simulink model "vikramsolarboost"  (R2017a)
settings: Solver=VariableStepAuto  StartTime=0.0  StopTime=1  MaxStep=1e-4  RelTol=1e-3
libraries: powerlib x11, powerlib_extras x2, simulink x2, powerlib_meascontrol x1
settings Model: Creator=Ankita Arora  LastModifiedBy=2
settings SolverCC: ZeroCrossAlgorithm=Adaptive
settings OptimizationCC: LifeSpan=inf
settings DebuggingCC: SFExecutionAtInitializationDiag=none

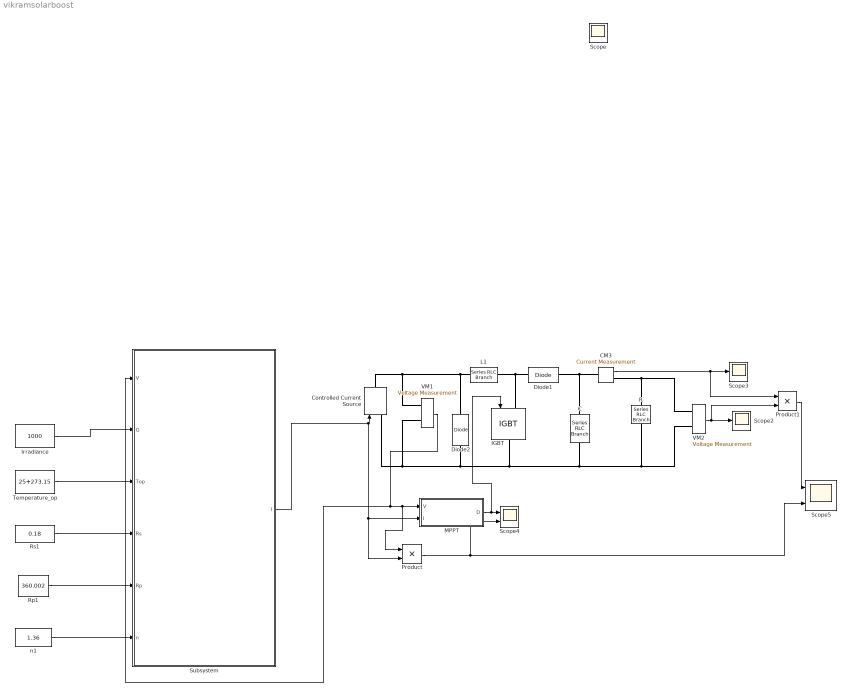
== system vikramsolarboost ==
  C : powerlib/Elements/Series RLC Branch  LConnTagsString=__new0  RConnTagsString=__new0  BranchType=C  Resistance=0.01  Inductance=1.0  SetiL0=off  InitialCurrent=0  Capacitance=3e-03  Setx0=off  InitialVoltage=200  Measurements=None
  CM3 : powerlib/Measurements/Current Measurement  Tag=PoWeRsYsTeMmEaSuReMeNt  PhasorSimulation=off  OutputType=Magnitude  PSBequivalent=0
  Controlled Current Source : powerlib/Electrical Sources/Controlled Current Source  Initialize=on  Source_Type=AC  Amplitude=0  Phase=0  Frequency=0  Measurements=None
  Diode1 : powerlib/Power Electronics/Diode  Ron=0.001  Lon=0  Vf=0.8  IC=0  UseSnubber=off  Rs=500  Cs=250e-9  Measurements=off
  Diode2 : powerlib/Power Electronics/Diode  Ron=0.001  Lon=0  Vf=0.8  IC=0  UseSnubber=off  Rs=500  Cs=250e-9  Measurements=off
  IGBT : powerlib/Power Electronics/IGBT  Ron=0.001  Lon=0  Vf=1  Tf=1e-6  Tt=2e-6  IC=0  Rs=1e5  Cs=inf  Measurements=off
  Irradiance : Constant  Value=1000
  L1 : powerlib/Elements/Series RLC Branch  LConnTagsString=__new0  RConnTagsString=__new0  BranchType=L  Resistance=1.0  Inductance=8.5e-03  SetiL0=off  InitialCurrent=0  Capacitance=1.0  Setx0=off  InitialVoltage=0  Measurements=None
  MPPT : Subsystem
  Product : Product  RndMeth=Zero
  Product1 : Product  RndMeth=Zero
  R : powerlib/Elements/Series RLC Branch  LConnTagsString=__new0  RConnTagsString=__new0  BranchType=R  Resistance=40  Inductance=1.0  SetiL0=off  InitialCurrent=0  Capacitance=1.0  Setx0=off  InitialVoltage=0  Measurements=None
  Rp1 : Constant  Value=360.002
  Rs1 : Constant  Value=0.18
  Scope : Scope
  Scope2 : Scope
  Scope3 : Scope
  Scope4 : Scope  NumInputPorts=2
  Scope5 : Scope  NumInputPorts=2
  Subsystem : Subsystem
  Temperature_op : Constant  Value=25+273.15
  VM1 : powerlib/Measurements/Voltage Measurement  Tag=PoWeRsYsTeMmEaSuReMeNt  PhasorSimulation=off  OutputType=Magnitude  PSBequivalent=0
  VM2 : powerlib/Measurements/Voltage Measurement  Tag=PoWeRsYsTeMmEaSuReMeNt  PhasorSimulation=off  OutputType=Magnitude  PSBequivalent=0
  n1 : Constant  Value=1.36
  wires:
  Temperature_op/1 -> Subsystem/3(Top)
  Rs1/1 -> Subsystem/4(Rs)
  Rp1/1 -> Subsystem/5(Rp)
  n1/1 -> Subsystem/6(n)
  CM3/1 -> Product1/1, Scope3/1
  VM2/1 -> Product1/2, Scope2/1
  Product/1 -> Scope5/2, Scope4/2
  MPPT/1(D) -> IGBT/1, Scope4/1
  Subsystem/1(I) -> MPPT/2(I), Product/2, Controlled Current Source/1
  Product1/1 -> Scope5/1
  VM1/1 -> Product/1, MPPT/1(V), Subsystem/1(V)
  Irradiance/1 -> Subsystem/2(G)
  connections:
  C/RConn1 -- VM2/LConn2 -- R/RConn1 -- IGBT/RConn1 -- Diode2/LConn1 -- Controlled Current Source/LConn1 -- VM1/LConn2
  Diode1/RConn1 -- CM3/LConn1 -- C/LConn1
  IGBT/LConn1 -- L1/RConn1 -- Diode1/LConn1
  VM2/LConn1 -- R/LConn1 -- CM3/RConn1
  VM1/LConn1 -- Diode2/RConn1 -- L1/LConn1 -- Controlled Current Source/RConn1

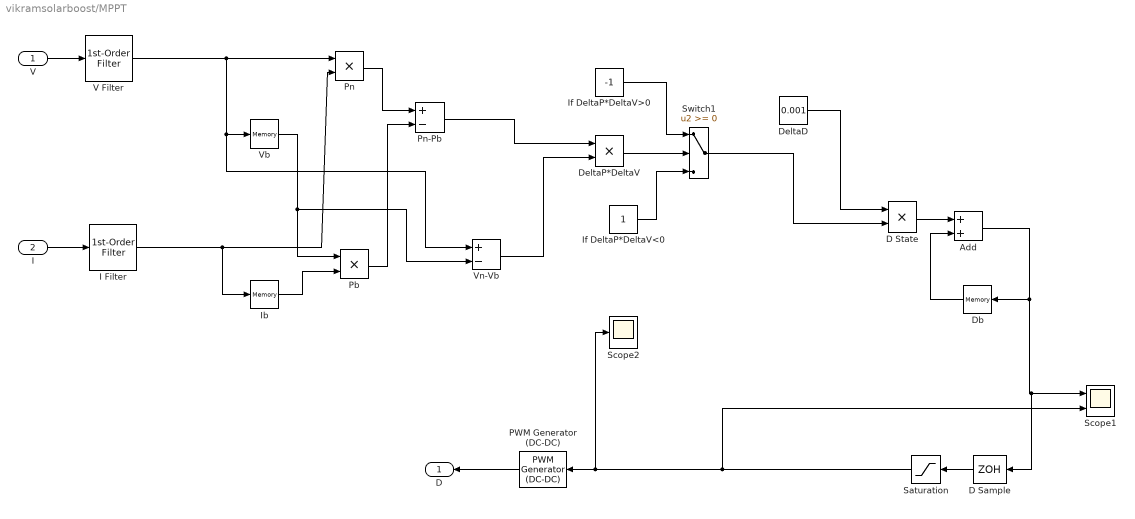
== system vikramsolarboost/MPPT ==
  V : Inport
  I : Inport  Port=2
  Add : Sum
  D Sample : ZeroOrderHold  SampleTime=1e-4
  D State : Product  RndMeth=Zero
  Db : Memory  InheritSampleTime=on  LinearizeAsDelay=on
  DeltaD : Constant  Value=0.001
  DeltaP*DeltaV : Product  RndMeth=Zero
  I Filter : powerlib_extras/Control  Blocks/1st-Order  Filter  FilterType=Lowpass  Tc=1e-3  Initialize=off  Vac_Init=[0.8 -25 60]  Vdc_Init=-0.4  PlotResponse=off  param1=[1 500 1]
  Ib : Memory  InheritSampleTime=on  LinearizeAsDelay=on
  If DeltaP*DeltaV<0 : Constant
  If DeltaP*DeltaV>0 : Constant  Value=-1
  PWM Generator (DC-DC) : powerlib_meascontrol/Pulse & Signal Generators/PWM Generator (DC-DC)  Fsw=5000  Ts=0
  Pb : Product  RndMeth=Zero
  Pn : Product  RndMeth=Zero
  Pn-Pb : Sum  Inputs=+-
  Saturation : Saturate  UpperLimit=0.8  LowerLimit=0
  Scope1 : Scope  NumInputPorts=2
  Scope2 : Scope
  Switch1 : Switch
  V Filter : powerlib_extras/Control  Blocks/1st-Order  Filter  FilterType=Lowpass  Tc=1e-3  Initialize=off  Vac_Init=[0.8 -25 60]  Vdc_Init=-0.4  PlotResponse=off  param1=[1 500 1]
  Vb : Memory  InheritSampleTime=on  LinearizeAsDelay=on
  Vn-Vb : Sum  Inputs=+-
  D : Outport
  wires:
  V/1 -> V Filter/1
  I/1 -> I Filter/1
  I Filter/1 -> Ib/1, Pn/2
  V Filter/1 -> Pn/1, Vb/1, Vn-Vb/1
  Ib/1 -> Pb/2
  Vb/1 -> Pb/1, Vn-Vb/2
  Pn/1 -> Pn-Pb/1
  Pb/1 -> Pn-Pb/2
  D State/1 -> Add/1
  Db/1 -> Add/2
  Pn-Pb/1 -> DeltaP*DeltaV/1
  Vn-Vb/1 -> DeltaP*DeltaV/2
  DeltaP*DeltaV/1 -> Switch1/2
  If DeltaP*DeltaV>0/1 -> Switch1/1
  If DeltaP*DeltaV<0/1 -> Switch1/3
  Switch1/1 -> D State/2
  DeltaD/1 -> D State/1
  Add/1 -> Db/1, D Sample/1, Scope1/1
  PWM Generator (DC-DC)/1 -> D/1
  Saturation/1 -> Scope1/2, PWM Generator (DC-DC)/1, Scope2/1
  D Sample/1 -> Saturation/1

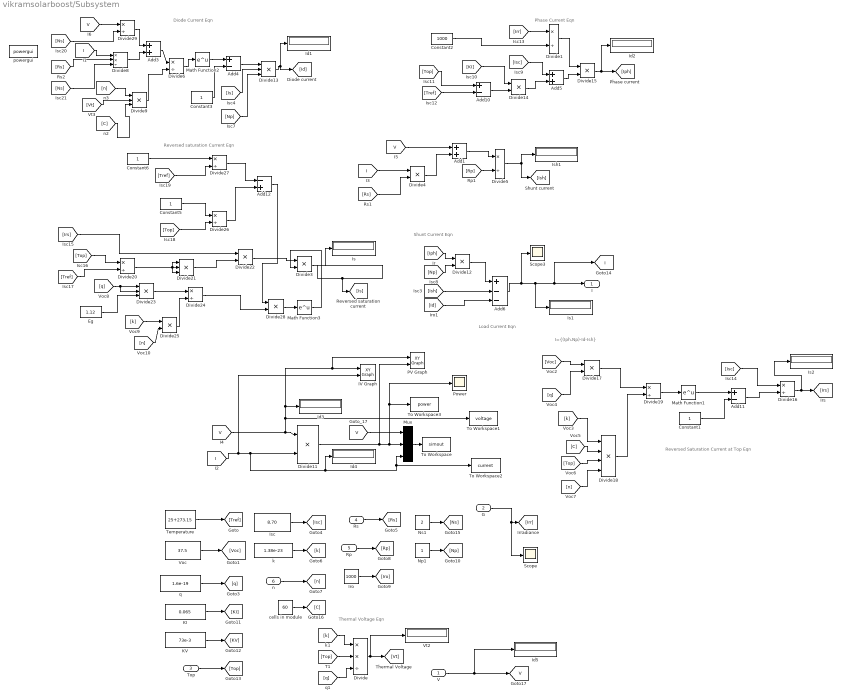
== system vikramsolarboost/Subsystem ==
  note: Diode Current Eqn
  note: Shunt Current Eqn
  note: Phase Current Eqn
  note: Reversed saturation Current Eqn
  note: Load Current Eqn
  note: I={(Iph.Np)-Id-Ish}
  note: Reversed Saturation Current at Top Eqn
  note: Thermal Voltage Eqn
  V : Inport
  G : Inport  Port=2
  Top : Inport  Port=3
  Rs : Inport  Port=4
  Rp : Inport  Port=5
  n : Inport  Port=6
  Add1 : Sum
  Add10 : Sum  Inputs=+-
  Add11 : Sum  Inputs=+-
  Add12 : Sum  Inputs=-+
  Add3 : Sum
  Add4 : Sum  Inputs=+-
  Add5 : Sum
  Add6 : Sum  Inputs=+--
  Constant{1,3,5..6} (4 alike) : Constant
  Constant2 : Constant  Value=1000
  Divide : Product  Inputs=**/
  Divide{1,5..6,16,19..20,24,26..27,29} (10 alike) : Product  Inputs=*/
  Divide{3..4,11..12,14..15,17,22,25,28} (10 alike) : Product  Inputs=**
  Divide{9,13,21,23} (4 alike) : Product  Inputs=***
  Divide18 : Product  Inputs=****
  Divide8 : Product  Inputs=**/
  Eg : Constant  Value=1.12
  IV Graph : simulink/Sinks/XY Graph  xmin=0  xmax=80  ymin=0  ymax=10  st=-1
  Id{1..5} (5 alike) : Display
  Iro : Constant  Value=1000
  Is : Display
  Is1 : Display
  Is2 : Display
  Isc : Constant  Value=8.70
  Ish1 : Display
  KI : Constant  Value=0.065
  KV : Constant  Value=73e-3
  Math Function1 : Math  SaturateOnIntegerOverflow=on
  Math Function2 : Math  SaturateOnIntegerOverflow=on
  Math Function3 : Math  SaturateOnIntegerOverflow=on
  Mux : Mux  Inputs=3
  Np1 : Constant
  Ns1 : Constant  Value=2
  PV Graph : simulink/Sinks/XY Graph  xmin=0  xmax=80  ymin=0  ymax=600  st=-1
  Power : Scope
  Scope : Scope
  Scope3 : Scope
  Temperature : Constant  Value=25+273.15
  To Workspace : ToWorkspace  VariableName=simout  SampleTime=-1
  To Workspace1 : ToWorkspace  VariableName=voltage  SampleTime=-1
  To Workspace2 : ToWorkspace  VariableName=current  SampleTime=-1
  To Workspace3 : ToWorkspace  VariableName=power  SampleTime=-1
  Voc : Constant  Value=37.5
  Vt2 : Display
      settings: Format=long_e
  cells in module : Constant  Value=60
  k : Constant  Value=1.38e-23
  powergui : powerlib/powergui  SimulationMode=Continuous  SampleTime=50e-6  frequency=60  Iterations=50  frequencyindice=0  Pbase=100e6  ErrMax=1e-4  UnitsV=kV  UnitsW=MW  buscounter=0  FunctionMessages=off  echomessages=off  EnableUseOfTLC=off  CurrentSourceSwitches=off  DisableSnubberDevices=off  DisableRonSwitches=off  DisableVfSwitches=off  DisplayEquations=off  SolverType=Tustin/Backward Euler (TBE)  Interpol=off  ExternalGateDelay=off  methode=off  Ts=100  x0status=blocks  SPID=on  SwTol=0  HookPort=off  RestoreLinks=warning  ResistiveCurrentMeasurement=off  Frange=[0:2:500]  Ylog=off  Xlog=on  ShowGrid=off  save=off  variable=ZData  structure=0  ZoomFFT=on  StartTime=0.0  cycles=1  DisplayStyle=1  fundamental=60  FreqAxis=off  MaxFrequency=1000  frequencyindicesteady=1  RmsSteady=1  display=off
  q : Constant  Value=1.6e-19
  I : Outport
  tag scope: I=global, V=global
  wires:
  [V] -> Add1/1
  [I] -> Divide4/1
  Divide4/1 -> Add1/2
  [Rs] -> Divide4/2
  Divide5/1 -> [Ish], Ish1/1
  Add1/1 -> Divide5/1
  [Rp] -> Divide5/2
  Add5/1 -> Divide15/2
  Divide15/1 -> [Iph], Id2/1
  Divide14/1 -> Add5/2
  [Top] -> Add10/1
  [KI] -> Divide14/1
  [Isc] -> Add5/1
  Add10/1 -> Divide14/2
  Divide13/1 -> [Id], Id1/1
  [n] -> Divide9/1
  [V] -> Divide29/1
  [I] -> Divide8/1
  Divide29/1 -> Add3/1
  [Rs] -> Divide8/2
  [Ns] -> Divide29/2
  Divide6/1 -> Math Function2/1
  Divide8/1 -> Add3/2
  [Ns] -> Divide8/3
  Constant3/1 -> Add4/2
  Math Function2/1 -> Add4/1
  Add3/1 -> Divide6/1
  [Np] -> Divide13/3
  [C] -> Divide9/3
  [Is] -> Divide13/2
  [Vt] -> Divide9/2
  Add4/1 -> Divide13/1
  Divide9/1 -> Divide6/2
  Math Function3/1 -> Divide3/2
  [n] -> Divide25/2
  Divide28/1 -> Math Function3/1
  Divide24/1 -> Divide28/2
  [k] -> Divide25/1
  Divide26/1 -> Add12/2
  Eg/1 -> Divide23/3
  [Tref] -> Divide27/2
  Divide3/1 -> Is/1, [Is]
  Constant5/1 -> Divide26/1
  Divide21/1 -> Divide22/2
  Divide25/1 -> Divide24/2
  Divide22/1 -> Divide3/1
  Divide20/1 -> Divide21/1, Divide21/2, Divide21/3
  [Irs] -> Divide22/1
  [Top] -> Divide26/2
  Divide23/1 -> Divide24/1
  [Tref] -> Divide20/2
  Divide27/1 -> Add12/1
  Add12/1 -> Divide28/1
  [q] -> Divide23/1, Divide23/2
  [Top] -> Divide20/1
  Constant6/1 -> Divide27/1
  Divide11/1 -> Mux/2, Power/1, To Workspace3/1, PV Graph/2
  [V] -> Mux/1
  Mux/1 -> To Workspace/1
  [I] -> Divide11/2, Mux/3, To Workspace2/1, Id4/1, IV Graph/2
  [V] -> Divide11/1, Id3/1, IV Graph/1, PV Graph/1, To Workspace1/1
  [Tref] -> Add10/2
  [Top] -> Divide18/3
  [n] -> Divide18/4
  Constant1/1 -> Add11/2
  Divide16/1 -> [Irs], Is2/1
  Math Function1/1 -> Add11/1
  Divide17/1 -> Divide19/1
  [q] -> Divide17/2
  Divide19/1 -> Math Function1/1
  [Isc] -> Divide16/1
  [C] -> Divide18/2
  Add11/1 -> Divide16/2
  [Voc] -> Divide17/1
  Divide18/1 -> Divide19/2
  [k] -> Divide18/1
  [Ish] -> Add6/2
  Add6/1 -> Scope3/1, Is1/1, I/1, [I]
  [Iph] -> Divide12/1
  [Np] -> Divide12/2
  Divide12/1 -> Add6/1
  [Id] -> Add6/3
  Isc/1 -> [Isc]
  [k] -> Divide/1
  k/1 -> [k]
  n/1 -> [n]
  Ns1/1 -> [Ns]
  [Top] -> Divide/2
  [q] -> Divide/3
  KV/1 -> [KV]
  KI/1 -> [KI]
  Temperature/1 -> [Tref]
  Np1/1 -> [Np]
  Rs/1 -> [Rs]
  Iro/1 -> [Iro]
  q/1 -> [q]
  G/1 -> [Irr], Scope/1
  Rp/1 -> [Rp]
  Divide/1 -> [Vt], Vt2/1
  cells in module/1 -> [C]
  Voc/1 -> [Voc]
  V/1 -> [V], Id5/1
  Top/1 -> [Top]
  [Irr] -> Divide1/1
  Divide1/1 -> Divide15/1
  Constant2/1 -> Divide1/2
